simulink model "carsim_experiment"  (R2017a)
settings: Solver=ode45  StartTime=0  StopTime=200  FixedStep=0.002  RelTol=1e-3  AbsTol=1e-6
PreLoadFcn:
  | addpath C:\MKZ
  | bus_definitions
settings Model: ExtModeTrigMode=oneshot  ExtModeArmWhenConnect=off  Creator=ywata  LastModifiedBy=User
settings DataIOCC: SaveFormat=Array  SignalLoggingSaveFormat=ModelDataLogs  SignalLoggingName=sigsOut
settings OptimizationCC: BlockReduction=off  BooleanDataType=off  LifeSpan=inf
settings DebuggingCC: SaveWithParameterizedLinksMsg=none  UnderspecifiedInitializationDetection=Classic  MergeDetectMultiDrivingBlocksExec=none  SignalResolutionControl=TryResolveAllWithWarning  MultiTaskDSMMsg=warning  MultiTaskCondExecSysMsg=none  FcnCallInpInsideContextMsg=warning  StateNameClashWarn=warning  SFUnexpectedBacktrackingDiag=warning  SFNoUnconditionalDefaultTransitionDiag=warning  SFExecutionAtInitializationDiag=none
settings HardwareCC: ProdBitPerPointer=32  ProdBitPerSizeT=32  ProdBitPerPtrDiffT=32  ProdLargestAtomicFloat=None  ProdIntDivRoundTo=Undefined  ProdEndianess=Unspecified  ProdWordSize=32  ProdHWDeviceType=32-bit Generic  TargetBitPerPointer=64  TargetBitPerSizeT=64  TargetBitPerPtrDiffT=64  TargetLongLongMode=on  TargetIntDivRoundTo=Zero  TargetEndianess=LittleEndian  TargetWordSize=64  TargetHWDeviceType=MATLAB Host  ProdEqTarget=off
settings ModelReferenceCC: UpdateModelReferenceTargets=Force  ModelReferenceNumInstancesAllowed=Single  PropagateSignalLabelsOutOfModel=off
settings ModelReferenceCC: ModelDependencies=|
  | lk_pcis_controller.m
  | road.m
settings RTWCC: TemplateMakefile=grt_vc.tmf
settings GRTTargetCC: TargetFcnLib=ansi_tfl_tmw.mat  TargetLangStandard=C89/C90 (ANSI)  GeneratePreprocessorConditionals=Disable all  CombineOutputUpdateFcns=off  GRTInterface=on
settings ConfigComp: CovMetricSettings=dw  CovHtmlReporting=on  CovSaveCumulativeToWorkspaceVar=on  CovSaveSingleToWorkspaceVar=on  CovExternalEMLEnable=off

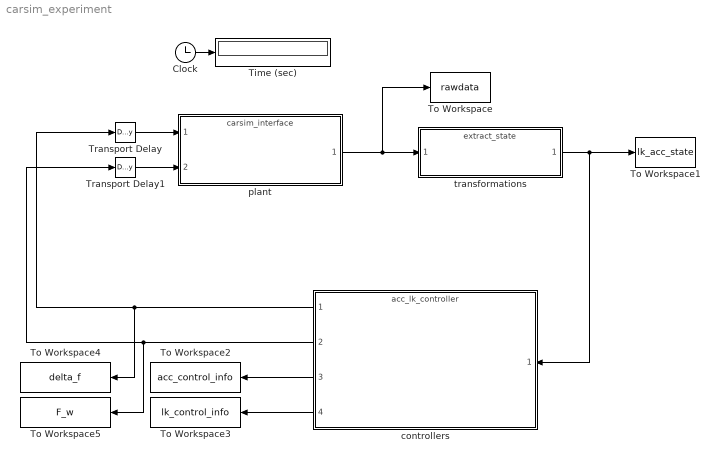
== system carsim_experiment ==
  Clock : Clock
  Time (sec) : Display
      settings: Format=bank  Decimation=100
  To Workspace : ToWorkspace  VariableName=rawdata  SaveFormat=Timeseries  SampleTime=-1
  To Workspace1 : ToWorkspace  VariableName=lk_acc_state  SaveFormat=Timeseries  SampleTime=-1
  To Workspace2 : ToWorkspace  VariableName=acc_control_info  SaveFormat=Timeseries  SampleTime=-1
  To Workspace3 : ToWorkspace  VariableName=lk_control_info  SaveFormat=Timeseries  SampleTime=-1
  To Workspace4 : ToWorkspace  VariableName=delta_f  SaveFormat=Timeseries  SampleTime=-1
  To Workspace5 : ToWorkspace  VariableName=F_w  SaveFormat=Timeseries  SampleTime=-1
  Transport Delay : TransportDelay  DelayTime=0.01
  Transport Delay1 : TransportDelay  DelayTime=0.01
  controllers : ModelReference  ModelNameDialog=acc_lk_controller  SimulationMode=Normal  ModelReferenceVersion=1.6
  plant : ModelReference  ModelNameDialog=carsim_interface  SimulationMode=Normal  ModelReferenceVersion=1.3
  transformations : ModelReference  ModelNameDialog=extract_state  SimulationMode=Normal  ModelReferenceVersion=1.3
  wires:
  Clock/1 -> Time (sec)/1
  plant/1 -> transformations/1, To Workspace/1
  Transport Delay/1 -> plant/1
  controllers/1 -> Transport Delay/1, To Workspace4/1
  Transport Delay1/1 -> plant/2
  controllers/2 -> To Workspace5/1, Transport Delay1/1
  transformations/1 -> controllers/1, To Workspace1/1
  controllers/3 -> To Workspace2/1
  controllers/4 -> To Workspace3/1
